simulink model "EV_longitude"  (R2024a)
settings: Solver=FixedStepAuto  StartTime=0  StopTime=inf  FixedStep=dt  RelTol=1e-3  EnableMultiTasking=on
InitFcn:
  | %open_system('EvReferenceApplication/Visualization/Performance and FE Scope');
  | dt = 0.001; %5e-5;
undefined symbols (not defined in the file): RealSimPara
libraries: autolibshared x1
settings Model: ModifiedByFormat=The MathWorks, Inc.  PauseTimes=0  Creator=The MathWorks, Inc.  LastModifiedBy=The MathWorks, Inc.
settings SolverCC: ZeroCrossAlgorithm=Adaptive  AlgebraicLoopSolver=TrustRegion  AutoInsertRateTranBlk=on  DecoupledContinuousIntegration=on  MinimalZcImpactIntegration=on
settings DataIOCC: SaveOutput=off  SignalLogging=off  DSMLogging=off  SaveTime=off
settings DebuggingCC: UnderspecifiedInitializationDetection=Classic  MergeDetectMultiDrivingBlocksExec=none  IgnoredZcDiagnostic=none  UnconnectedInputMsg=warning  UnconnectedOutputMsg=warning  UnconnectedLineMsg=warning  PregeneratedLibrarySubsystemCodeDiagnostic=none  ArithmeticOperatorsInVariantConditions=warning
settings ModelReferenceCC: UpdateModelReferenceTargets=IfOutOfDate  EnableRefExpFcnMdlSchedulingChecks=on  ModelReferenceMinAlgLoopOccurrences=on  PropagateSignalLabelsOutOfModel=off
settings SFSimCC: SimUseLocalCustomCode=off
settings RTWCC: RTWUseLocalCustomCode=off  GPUComputeCapability=3.5
settings CodeAppCC: StateflowObjectComments=on
settings GRTTargetCC: TargetLangStandard=C89/C90 (ANSI)
settings ConfigComp: CovMetricSettings=dsw  CovSaveCumulativeToWorkspaceVar=on  CovSaveSingleToWorkspaceVar=on  CovExternalEMLEnable=off

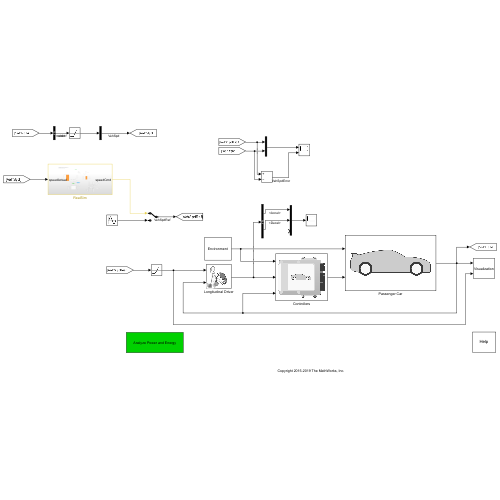
[thumbnail: Simulink's stored preview of the top-level diagram]
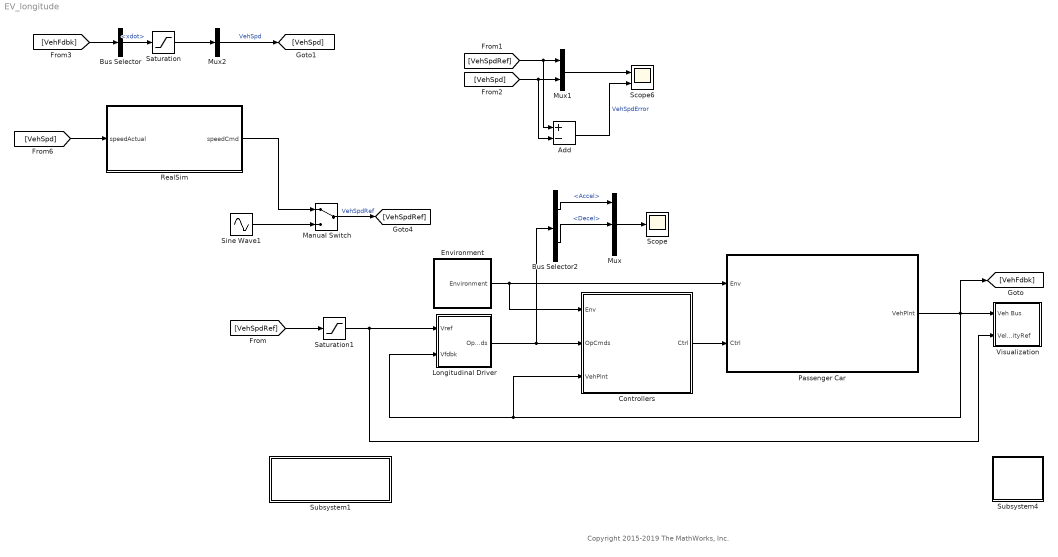
== system EV_longitude ==
  note: Copyright 2015-2019 The MathWorks, Inc.
  Add : Sum  Inputs=+-
  Bus Selector : BusSelector  OutputSignals=Veh.xdot
  Bus Selector2 : BusSelector  OutputSignals=Accel,Decel
  Controllers : Subsystem
      mask Display: image('SystemControllers.png','center')
  Environment : Subsystem
      mask Display: disp('Environment')
  Longitudinal Driver : Subsystem  Variant=on  VariantControlMode=label  VariantControl=Variant1  LabelModeActiveChoice=0  mask{tau=0.03, L=4, Kpt=10000}
      mask prompts: tau "Driver response time, tau [s]"; L "Preview distance, L [m]:"; Kpt "Effective vehicle total tractive force, Kpt [N]:"
      mask Display:
      | if strcmp('1',get_param(gcb,'ActiveVariant'))
      |     disp('Open Loop')
      | else
      |     image('LongitudinalDriver.png','center');
      | end
  Manual Switch : ManualSwitch
  Mux : Mux  Inputs=3
  Mux1 : Mux  Inputs=2
  Mux2 : Mux  Inputs=1
  Passenger Car : Subsystem
      mask Display: image('PassengerVehicle.png','center')
  RealSim : Subsystem
  Saturation : Saturate  UpperLimit=Inf  LowerLimit=0.0
  Saturation1 : Saturate  UpperLimit=Inf  LowerLimit=0.0
  Scope : Scope
  Scope6 : Scope  NumInputPorts=2
  Sine Wave1 : Sin  Bias=10  SampleTime=0
  Subsystem1 : Subsystem
      settings: OpenFcn=edit GenerateEnergyReport
      mask Display: disp('Analyze Power and Energy')
  Subsystem4 : Subsystem
      settings: OpenFcn=helpview([docroot,'/toolbox/autoblks/helptargets.map'], 'ev_refapp')
      mask Display: disp('Help')
  Visualization : Subsystem
      mask Display: disp('Visualization')
  wires:
  [VehSpdRef] -> Saturation1/1
  Environment/1(Environment) -> Controllers/1(Env), Passenger Car/1(Env)
  Controllers/1(Ctrl) -> Passenger Car/2(Ctrl)
  Mux1/1 -> Scope6/1
  Manual Switch/1 -> [VehSpdRef]  "VehSpdRef"
  [VehSpd] -> Add/2, Mux1/2
  Sine Wave1/1 -> Manual Switch/2
  RealSim/1(speedCmd) -> Manual Switch/1
  [VehSpdRef] -> Add/1, Mux1/1
  [VehSpd] -> RealSim/1(speedActual)
  Add/1 -> Scope6/2  "VehSpdError"
  Bus Selector/1 -> Saturation/1  "<xdot>"
  [VehFdbk] -> Bus Selector/1
  Passenger Car/1(VehPlnt) -> [VehFdbk], Longitudinal Driver/2("Vfdbk "), Controllers/3(VehPlnt), Visualization/1(Veh Bus)
  Bus Selector2/2 -> Mux/2  "<Decel>"
  Longitudinal Driver/1(" OpCmds") -> Bus Selector2/1, Controllers/2(OpCmds)
  Mux/1 -> Scope/1
  Bus Selector2/1 -> Mux/1  "<Accel>"
  Mux2/1 -> [VehSpd]  "VehSpd"
  Saturation/1 -> Mux2/1
  Saturation1/1 -> Visualization/2(VelocityRef), Longitudinal Driver/1("Vref ")

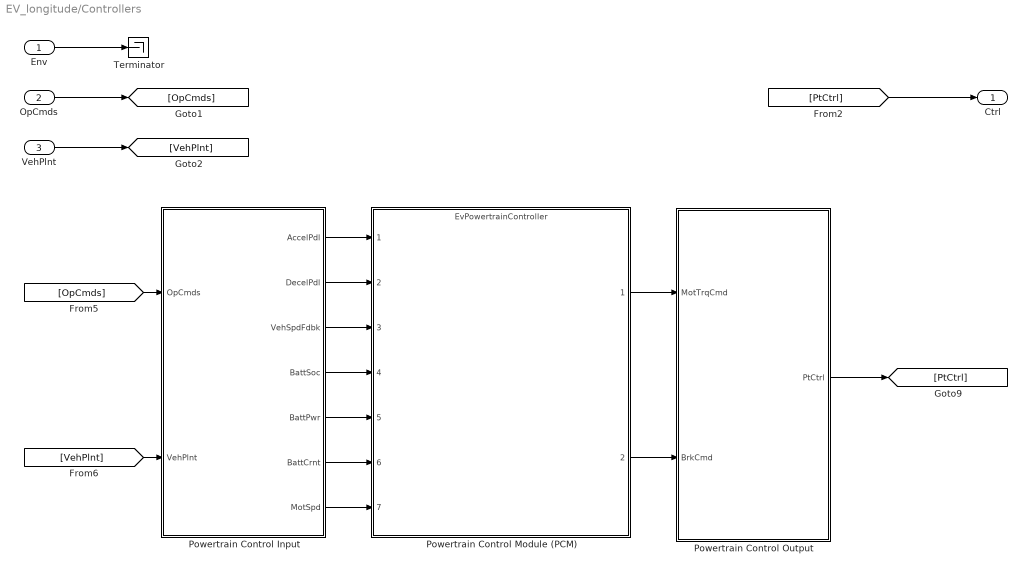
== system EV_longitude/Controllers ==
  Env : Inport
  OpCmds : Inport  Port=2
  VehPlnt : Inport  Port=3
  Powertrain Control Input : Subsystem
  Powertrain Control Module (PCM) : ModelReference  ModelNameDialog=EvPowertrainController.slx  SimulationMode=Normal  ModelReferenceVersion=1.415
  Powertrain Control Output : Subsystem
  Terminator : Terminator
  Ctrl : Outport  VectorParamsAs1DForOutWhenUnconnected=off
  wires:
  [PtCtrl] -> Ctrl/1
  Env/1 -> Terminator/1
  [OpCmds] -> Powertrain Control Input/1(OpCmds)
  Powertrain Control Output/1(PtCtrl) -> [PtCtrl]
  [VehPlnt] -> Powertrain Control Input/2(VehPlnt)
  VehPlnt/1 -> [VehPlnt]
  OpCmds/1 -> [OpCmds]
  Powertrain Control Input/4(BattSoc) -> Powertrain Control Module (PCM)/4
  Powertrain Control Input/3(VehSpdFdbk) -> Powertrain Control Module (PCM)/3
  Powertrain Control Input/2(DecelPdl) -> Powertrain Control Module (PCM)/2
  Powertrain Control Input/1(AccelPdl) -> Powertrain Control Module (PCM)/1
  Powertrain Control Input/5(BattPwr) -> Powertrain Control Module (PCM)/5
  Powertrain Control Input/6(BattCrnt) -> Powertrain Control Module (PCM)/6
  Powertrain Control Input/7(MotSpd) -> Powertrain Control Module (PCM)/7
  Powertrain Control Module (PCM)/1 -> Powertrain Control Output/1(MotTrqCmd)
  Powertrain Control Module (PCM)/2 -> Powertrain Control Output/2(BrkCmd)

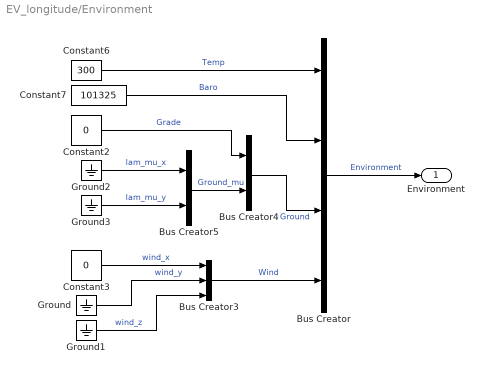
== system EV_longitude/Environment ==
  Bus Creator : BusCreator  Inputs=4
  Bus Creator3 : BusCreator  Inputs=3
  Bus Creator4 : BusCreator  Inputs=2
  Bus Creator5 : BusCreator  Inputs=2
  Constant2 : Constant  Value=0
  Constant3 : Constant  Value=0
  Constant6 : Constant  Value=300
  Constant7 : Constant  Value=101325
  Ground{,1..3} (4 alike) : Ground
  Environment : Outport  VectorParamsAs1DForOutWhenUnconnected=off
  wires:
  Ground2/1 -> Bus Creator5/1  "lam_mu_x"
  Ground3/1 -> Bus Creator5/2  "lam_mu_y"
  Bus Creator5/1 -> Bus Creator4/2  "Ground_mu"
  Bus Creator4/1 -> Bus Creator/3  "Ground"
  Bus Creator3/1 -> Bus Creator/4  "Wind"
  Constant3/1 -> Bus Creator3/1  "wind_x"
  Ground/1 -> Bus Creator3/2  "wind_y"
  Ground1/1 -> Bus Creator3/3  "wind_z"
  Constant6/1 -> Bus Creator/1  "Temp"
  Constant2/1 -> Bus Creator4/1  "Grade"
  Bus Creator/1 -> Environment/1  "Environment"
  Constant7/1 -> Bus Creator/2  "Baro"

== system EV_longitude/Longitudinal Driver ==
  note: To switch variants, right-click on this subsystem (from one level above) and chose:
      | Variant, Active choice, <your selection>
  "Vref " : Inport
  "Vfdbk " : Inport  Port=2
  Longitudinal Driver : Subsystem  VariantControl=0
      mask Display: image('LongitudinalDriver.png', 'center')
  Open Loop : Subsystem  VariantControl=1
      mask Display: disp('Open Loop')
  " OpCmds" : Outport  VectorParamsAs1DForOutWhenUnconnected=off

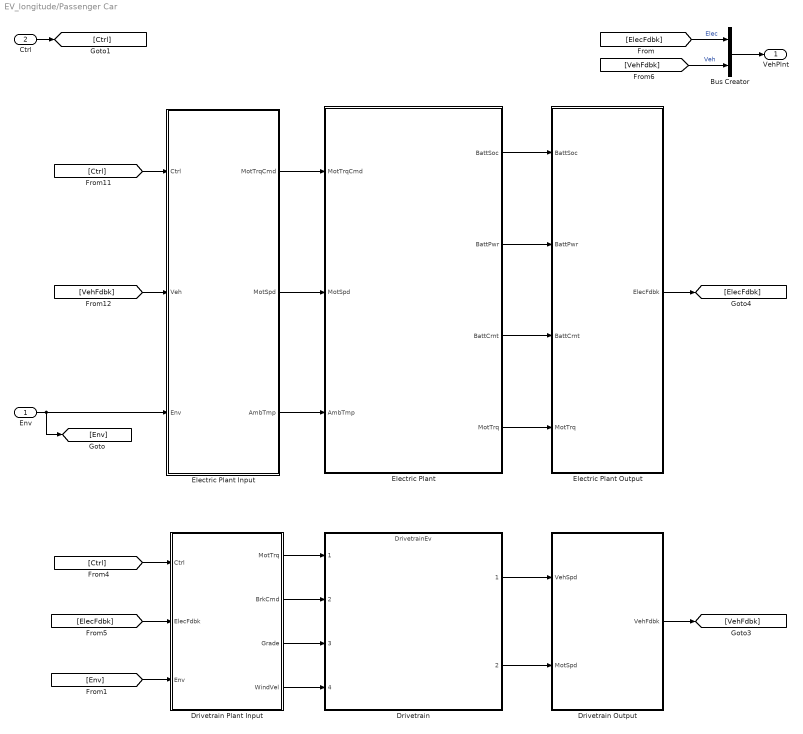
== system EV_longitude/Passenger Car ==
  Env : Inport
  Ctrl : Inport  Port=2
  Bus Creator : BusCreator  Inputs=2
  Drivetrain : ModelReference  ModelNameDialog=DrivetrainEv.slx  SimulationMode=Normal  ModelReferenceVersion=1.457
  Drivetrain Output : Subsystem
  Drivetrain Plant Input : Subsystem
  Electric Plant : Subsystem
  Electric Plant Input : Subsystem
  Electric Plant Output : Subsystem
  VehPlnt : Outport  VectorParamsAs1DForOutWhenUnconnected=off
  wires:
  Ctrl/1 -> [Ctrl]
  Env/1 -> [Env], Electric Plant Input/3(Env)
  [Ctrl] -> Drivetrain Plant Input/1(Ctrl)
  Bus Creator/1 -> VehPlnt/1
  [VehFdbk] -> Bus Creator/2  "Veh"
  Drivetrain Output/1(VehFdbk) -> [VehFdbk]
  Electric Plant Output/1(ElecFdbk) -> [ElecFdbk]
  [ElecFdbk] -> Bus Creator/1  "Elec"
  [Ctrl] -> Electric Plant Input/1(Ctrl)
  [ElecFdbk] -> Drivetrain Plant Input/2(ElecFdbk)
  [VehFdbk] -> Electric Plant Input/2(Veh)
  Drivetrain Plant Input/2(BrkCmd) -> Drivetrain/2
  Drivetrain Plant Input/1(MotTrq) -> Drivetrain/1
  Drivetrain/2 -> Drivetrain Output/2(MotSpd)
  Drivetrain/1 -> Drivetrain Output/1(VehSpd)
  Electric Plant Input/1(MotTrqCmd) -> Electric Plant/1(MotTrqCmd)
  Electric Plant Input/2(MotSpd) -> Electric Plant/2(MotSpd)
  Electric Plant/1(BattSoc) -> Electric Plant Output/1(BattSoc)
  Electric Plant/2(BattPwr) -> Electric Plant Output/2(BattPwr)
  Electric Plant/3(BattCrnt) -> Electric Plant Output/3(BattCrnt)
  Electric Plant/4(MotTrq) -> Electric Plant Output/4(MotTrq)
  Electric Plant Input/3(AmbTmp) -> Electric Plant/3(AmbTmp)
  [Env] -> Drivetrain Plant Input/3(Env)
  Drivetrain Plant Input/3(Grade) -> Drivetrain/3
  Drivetrain Plant Input/4(WindVel) -> Drivetrain/4

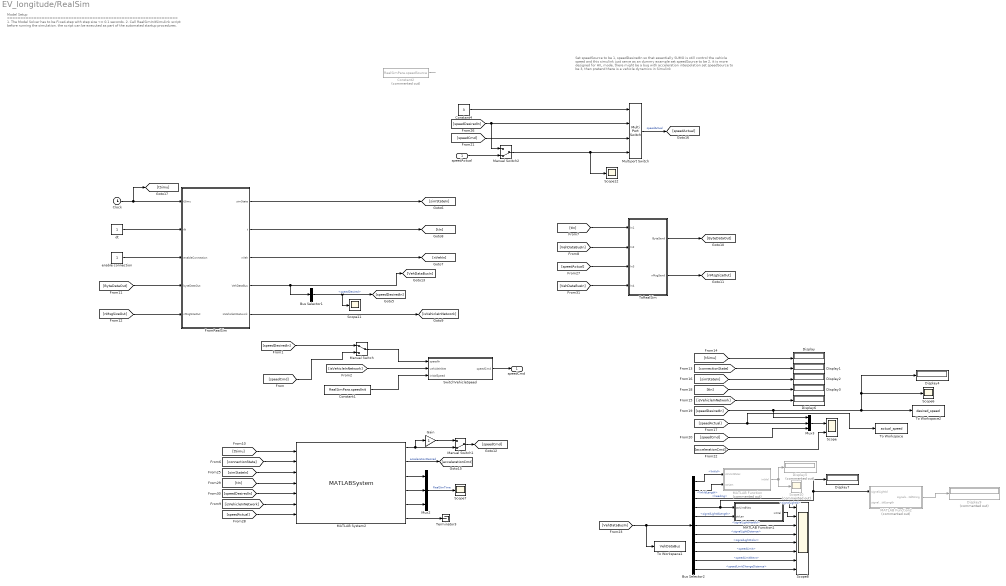
== system EV_longitude/RealSim ==
  note: Model Setup
      | ================================================================
      | 1. The Model Solver has to be Fixed-step with step size <= 0.1 seconds.
      | 2. Call RealSimInitSimulink script before running the simulation. the script can be executed as part of the automated startup procedures.
  note: Set speedSource to be 1, speedDesiredIn so that essentially SUMO is still control the vehicle speed and this simulink just serve as an dummy example
      |
      | set speedSource to be 2, it is more designed for HIL mode, there might be a bug with acceleration interpolation
      |
      | set speedSource to be 3, then pretend there is a vehicle dynamics in Simulink
  speedActual : Inport
  Bus Selector1 : BusSelector  OutputSignals=speedDesired
  Bus Selector2 : BusSelector  OutputSignals=linkId,linkIdLength,heading,signalLightId,signalLightIdLength,signalLightHeadId,signalLightDistance,signalLightColor,speedLimit,speedLimitNext,speedLimitChangeDistance
  Clock : Clock
  Constant1 : Constant  Value=RealSimPara.speedInit
  Constant2 : Constant  Commented=on  Value=RealSimPara.speedSource
  Constant4 : Constant  Value=3
  Display{,1..4,6..7} (7 alike) : Display
  Display5 : Display  Commented=on
  Display9 : Display  Commented=on
  FromRealSim : Subsystem
  Gain : Gain
  MATLAB Function : MATLAB Function  Commented=on  TreatAsAtomicUnit=on
  MATLAB Function1 : MATLAB Function  TreatAsAtomicUnit=on
  MATLAB Function2 : MATLAB Function  Commented=on  TreatAsAtomicUnit=on  SystemSampleTime=0.001
  MATLAB System2 : MATLABSystem  System=RealSimInterpSpeed  initialSpeed=RealSimPara.speedInit  speedLookAheadHorizon=RealSimPara.tLookahead  speedUpperBound=30  smoothWindow=RealSimPara.smoothWindow  SimulateUsing=Code generation
      mask Type: RealSimInterpSpeed
      mask Display:
      | disp('RealSimInterpSpeed');
      | port_label('input',1,'simulationTime');
      | port_label('input',2,'connectionState');
      | port_label('input',3,'simState');
      | port_label('input',4,'timeReceive');
      | port_label('input',5,'speedReceive');
      | port_label('input',6,'isVehicleInNetwork');
      | port_label('input',7,'speedActual');
      | port_label('output',1,'speedLookAhead');
      | port_label('output',2,'accelerationDesired');
      | port_label('output',3,'timeSimulator');
      | port_label('output',4,'timeStepSimulator');
      | port_label('output',5,'timeStepTrigger');
      | port_label('output',6,'RealSimDelay');
  Manual Switch : ManualSwitch
  Manual Switch1 : ManualSwitch  CurrentSetting=0
  Manual Switch2 : ManualSwitch  CurrentSetting=0
  Multiport Switch : MultiPortSwitch  SaturateOnIntegerOverflow=off  InputSameDT=off
  Mux2 : Mux  Inputs=3
  Mux3 : Mux  Inputs=3
  Scope : Scope  NumInputPorts=2
  Scope10 : Scope  Commented=on
  Scope{6..7,11..12} (4 alike) : Scope
  Scope8 : Scope  NumInputPorts=8
  SwitchVehicleSpeed : Subsystem
  Terminator3 : Terminator
  To Workspace : ToWorkspace  VariableName=actual_speed  SaveFormat=Timeseries  SampleTime=1
  To Workspace1 : ToWorkspace  VariableName=VehDataBus  SaveFormat=Timeseries  SampleTime=-1
  To Workspace2 : ToWorkspace  VariableName=desired_speed  SaveFormat=Timeseries  SampleTime=1
  ToRealSim : Subsystem
  dt : Constant
  enable connection : Constant
  speedCmd : Outport
  wires:
  [tSimu] -> Display/1
  Bus Selector2/5 -> MATLAB Function1/2(strLen)  "<signalLightIdLength>"
  [simStateIn] -> MATLAB System2/3
  [isVehicleInNetwork] -> Display6/1
  [ByteDataOut] -> FromRealSim/4(byteDataOut)
  MATLAB System2/5 -> Mux2/3
  [VehDataBusIn] -> To Workspace1/1, Bus Selector2/1
  MATLAB System2/1 -> Gain/1, Manual Switch1/2
  [speedCmd] -> Multiport Switch/3
  Mux2/1 -> Scope7/1  "RealSimTime"
  [tSimu] -> MATLAB System2/1
  Gain/1 -> Manual Switch1/1
  Bus Selector1/1 -> Scope11/1, [speedDesiredIn]  "<speedDesired>"
  Bus Selector2/9 -> Scope8/6  "<speedLimit>"
  [speedDesiredIn] -> Display4/1, Scope6/1, To Workspace2/1, Mux3/1
  Bus Selector2/4 -> Display7/1, MATLAB Function2/1(signalLightId), MATLAB Function1/1(strUint8Vec)  "<signalLightId>"
  MATLAB System2/3 -> Mux2/1
  dt/1 -> FromRealSim/2(dt)
  Bus Selector2/10 -> Scope8/7  "<speedLimitNext>"
  FromRealSim/4(VehDataBus) -> Bus Selector1/1, [VehDataBusIn]
  enable connection/1 -> FromRealSim/3(enableConnection)
  MATLAB Function/1(intVal) -> Scope10/1, Display5/1
  [speedDesiredIn] -> MATLAB System2/5
  [nMsgSizeOut] -> FromRealSim/5(nMsgSizeOut)
  Bus Selector2/11 -> Scope8/8  "<speedLimitChangeDistance>"
  [speedDesiredIn] -> Manual Switch2/1, Multiport Switch/2
  [speedActual] -> MATLAB System2/7
  FromRealSim/3(nVeh) -> [nVehIn]
  [speedActual] -> To Workspace/1, Mux3/2
  [connectionState] -> Display1/1
  Clock/1 -> FromRealSim/1(tSimu), [tSimu]
  [tIn] -> Display3/1
  Bus Selector2/7 -> Scope8/4  "<signalLightDistance>"
  MATLAB System2/4 -> Mux2/2
  Bus Selector2/8 -> Scope8/5  "<signalLightColor>"
  Manual Switch2/1 -> Scope12/1, Multiport Switch/4
  [connectionState] -> MATLAB System2/2
  MATLAB System2/6 -> Terminator3/1
  Bus Selector2/1 -> MATLAB Function/1(strUint8Vec)  "<linkId>"
  [tIn] -> ToRealSim/1(In1)
  MATLAB System2/2 -> [accelerationCmd]  "accelerationDesired"
  MATLAB Function2/1(signalLightIdString) -> Display9/1
  Bus Selector2/2 -> MATLAB Function/2(strLen)  "<linkIdLength>"
  [tIn] -> MATLAB System2/4
  [speedCmd] -> Mux3/3
  Constant4/1 -> Multiport Switch/1
  Manual Switch1/1 -> [speedCmd]
  ToRealSim/2(nMsgSend) -> [nMsgSizeOut]
  FromRealSim/1(simState) -> [simStateIn]
  [speedActual] -> ToRealSim/3(In3)
  FromRealSim/2(t) -> [tIn]
  FromRealSim/5(isVehicleInNetwork) -> [isVehicleInNetwork]
  [accelerationCmd] -> Scope/2
  [VehDataBusIn] -> ToRealSim/2(In2)
  Multiport Switch/1 -> [speedActual]  "speedActual"
  Bus Selector2/6 -> Scope8/3  "<signalLightHeadId>"
  [VehDataBusIn] -> ToRealSim/4(In4)
  ToRealSim/1(ByteSend) -> [ByteDataOut]
  MATLAB Function1/1(intVal) -> Scope8/2
  Bus Selector2/3 -> Scope8/1  "<heading>"
  [isVehicleInNetwork] -> MATLAB System2/6
  Mux3/1 -> Scope/1
  [simStateIn] -> Display2/1
  ? -> MATLAB Function2/2(signalLightIdLength)
  Constant2/1 -> ?
  [speedCmd] -> Manual Switch/2
  [speedDesiredIn] -> Manual Switch/1
  speedActual/1 -> Manual Switch2/2
  Constant1/1 -> SwitchVehicleSpeed/3(initialSpeed)
  [isVehicleInNetwork] -> SwitchVehicleSpeed/2(vehicleInNet)
  SwitchVehicleSpeed/1(speedCmd) -> speedCmd/1
  Manual Switch/1 -> SwitchVehicleSpeed/1(speedIn)

== system EV_longitude/Subsystem1 ==

== system EV_longitude/Subsystem4 ==

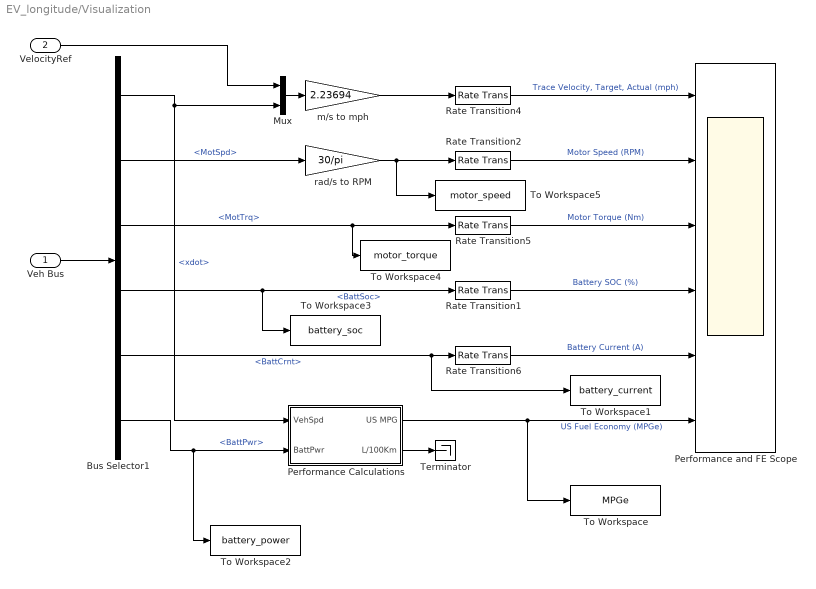
== system EV_longitude/Visualization ==
  Veh Bus : Inport
  VelocityRef : Inport  Port=2
  Bus Selector1 : BusSelector  OutputSignals=Veh.xdot,Veh.MotSpd,Elec.MotTrq,Elec.BattSoc,Elec.BattCrnt,Elec.BattPwr
  Mux : Mux  Inputs=2
  Performance Calculations : Subsystem
  Performance and FE Scope : Scope  NumInputPorts=6
  Rate Transition{1..2,4..6} (5 alike) : RateTransition  Deterministic=off
  Terminator : Terminator
  To Workspace : ToWorkspace  VariableName=MPGe  SaveFormat=Timeseries  SampleTime=1
  To Workspace1 : ToWorkspace  VariableName=battery_current  SaveFormat=Timeseries  SampleTime=1
  To Workspace2 : ToWorkspace  VariableName=battery_power  SaveFormat=Timeseries  SampleTime=1
  To Workspace3 : ToWorkspace  VariableName=battery_soc  SaveFormat=Timeseries  SampleTime=1
  To Workspace4 : ToWorkspace  VariableName=motor_torque  SaveFormat=Timeseries  SampleTime=1
  To Workspace5 : ToWorkspace  VariableName=motor_speed  SaveFormat=Timeseries  SampleTime=1
  m/s to mph : Gain  Gain=2.23694
  rad/s to RPM : Gain  Gain=30/pi
  wires:
  Veh Bus/1 -> Bus Selector1/1
  Bus Selector1/1 -> Performance Calculations/1(VehSpd), Mux/2  "<xdot>"
  Mux/1 -> m/s to mph/1
  Performance Calculations/1(US MPG) -> To Workspace/1, Performance and FE Scope/6  "US Fuel Economy (MPGe)"
  Performance Calculations/2(L/100Km) -> Terminator/1
  m/s to mph/1 -> Rate Transition4/1
  Bus Selector1/4 -> To Workspace3/1, Rate Transition1/1  "<BattSoc>"
  VelocityRef/1 -> Mux/1
  Rate Transition1/1 -> Performance and FE Scope/4  "Battery SOC (%)"
  Rate Transition2/1 -> Performance and FE Scope/2  "Motor Speed (RPM)"
  Rate Transition4/1 -> Performance and FE Scope/1  "Trace Velocity, Target, Actual (mph)"
  Bus Selector1/2 -> rad/s to RPM/1  "<MotSpd>"
  Bus Selector1/6 -> To Workspace2/1, Performance Calculations/2(BattPwr)  "<BattPwr>"
  rad/s to RPM/1 -> To Workspace5/1, Rate Transition2/1
  Bus Selector1/3 -> To Workspace4/1, Rate Transition5/1  "<MotTrq>"
  Rate Transition5/1 -> Performance and FE Scope/3  "Motor Torque (Nm)"
  Rate Transition6/1 -> Performance and FE Scope/5  "Battery Current (A)"
  Bus Selector1/5 -> To Workspace1/1, Rate Transition6/1  "<BattCrnt>"

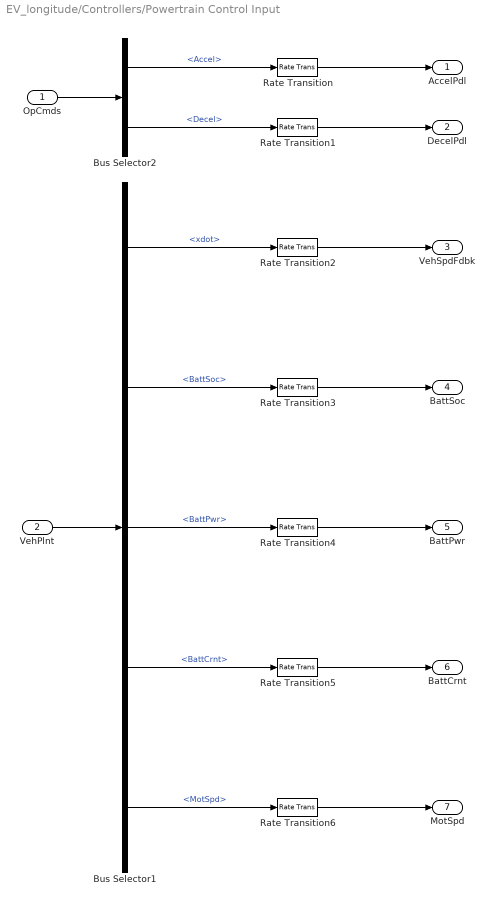
== system EV_longitude/Controllers/Powertrain Control Input ==
  OpCmds : Inport
  VehPlnt : Inport  Port=2
  Bus Selector1 : BusSelector  OutputSignals=Veh.xdot,Elec.BattSoc,Elec.BattPwr,Elec.BattCrnt,Veh.MotSpd
  Bus Selector2 : BusSelector  OutputSignals=Accel,Decel
  Rate Transition{,1..6} (7 alike) : RateTransition  Deterministic=off
  AccelPdl : Outport  VectorParamsAs1DForOutWhenUnconnected=off
  DecelPdl : Outport  Port=2  VectorParamsAs1DForOutWhenUnconnected=off
  VehSpdFdbk : Outport  Port=3  VectorParamsAs1DForOutWhenUnconnected=off
  BattSoc : Outport  Port=4  VectorParamsAs1DForOutWhenUnconnected=off
  BattPwr : Outport  Port=5  VectorParamsAs1DForOutWhenUnconnected=off
  BattCrnt : Outport  Port=6  VectorParamsAs1DForOutWhenUnconnected=off
  MotSpd : Outport  Port=7  VectorParamsAs1DForOutWhenUnconnected=off
  wires:
  OpCmds/1 -> Bus Selector2/1
  VehPlnt/1 -> Bus Selector1/1
  Bus Selector2/1 -> Rate Transition/1  "<Accel>"
  Bus Selector2/2 -> Rate Transition1/1  "<Decel>"
  Bus Selector1/1 -> Rate Transition2/1  "<xdot>"
  Bus Selector1/2 -> Rate Transition3/1  "<BattSoc>"
  Bus Selector1/3 -> Rate Transition4/1  "<BattPwr>"
  Bus Selector1/4 -> Rate Transition5/1  "<BattCrnt>"
  Bus Selector1/5 -> Rate Transition6/1  "<MotSpd>"
  Rate Transition/1 -> AccelPdl/1
  Rate Transition1/1 -> DecelPdl/1
  Rate Transition2/1 -> VehSpdFdbk/1
  Rate Transition3/1 -> BattSoc/1
  Rate Transition4/1 -> BattPwr/1
  Rate Transition5/1 -> BattCrnt/1
  Rate Transition6/1 -> MotSpd/1

== system EV_longitude/Controllers/Powertrain Control Output ==
  MotTrqCmd : Inport
  BrkCmd : Inport  Port=2
  Bus Creator : BusCreator  Inputs=2
  PtCtrl : Outport  VectorParamsAs1DForOutWhenUnconnected=off
  wires:
  BrkCmd/1 -> Bus Creator/2  "BrkCmd"
  Bus Creator/1 -> PtCtrl/1  "PtCtrl"
  MotTrqCmd/1 -> Bus Creator/1  "MotTrqCmd"

== system EV_longitude/Longitudinal Driver/Longitudinal Driver ==
  Vref : Inport
  Vfdbk : Inport  Port=2
  Bus Selector : BusSelector  OutputSignals=Veh.xdot
  Ground : Ground
  Longitudinal Driver Model : autolibshared/Longitudinal Driver  extAccelOvr=off  extDecelOvr=off  extAccelHld=off  extDecelHld=off  extAccelZero=off  extDecelZero=off  cntrlType=Predictive  shftType=Reverse, Neutral, Drive  velUnits=m/s  gearOut=off  Kp=1  Ki=1  Kff=0  Kg=0  VehVelVec=[0 100]  KffVec=[.1 .1]  KpVec=[10 10]  KiVec=[5 5]  KgVec=[0 0]  m=1500  Kpt=Kpt  tau=tau  L=L  aR=160  bR=1  cR=0.36  g=9.81  vnom=1  Kaw=0  tauerr=0  tauPt=2  GearInit=0  tShift=.1  pdlVec=[0.1 0.4 0.5 0.9]  upShftTbl=[-1 12.9375 26.4375 39.9375 51.18749999999999 62.4375 72.84375 83.25;-1 16.3125 29.8125 43.3125 54.5624 65.8125 76.78125 87.75;-1 19.6875 33.1875 46.68749999999999 57.9375 69.1875 80.71875 92.25;-1 33 52.5 77.25 100.5 138.75 161.875 185]  dwnShftTbl=[1 9.5625 23.0625 36.5625 47.8125 59.0625 68.90625 78.75;1 12.9375 26.4375 39.9375 51.18749999999999 62.4375 72.84375 83.25;1 16.3125 29.8125 43.3125 54.562499 65.8125 76.78125 87.75;1 19.6875 33.1875 46.68749999999999 57.9375 69.1875 80.71875 92.25]  tClutch=.5  tRev=.5  tPark=120  aMode=1  UpGearVec="[0  1  2  3  4  5  6  7]"  DownGearVec="[1  2  3  4  5  6  7  8]"
  Terminator : Terminator
  Terminator1 : Terminator
  OpCmds : Outport  VectorParamsAs1DForOutWhenUnconnected=off
  wires:
  Bus Selector/1 -> Longitudinal Driver Model/2  "<xdot>"
  Vref/1 -> Longitudinal Driver Model/1  "xdotref"
  Vfdbk/1 -> Bus Selector/1
  Longitudinal Driver Model/2 -> Terminator/1  "Acc"
  Longitudinal Driver Model/3 -> Terminator1/1  "Dec"
  Ground/1 -> Longitudinal Driver Model/3
  Longitudinal Driver Model/1 -> OpCmds/1  "Info"

== system EV_longitude/Longitudinal Driver/Open Loop ==
  note: This subsystem is provided to disable the driver subsystem and expose the driver interface.
      |
      | The interface can:
      | - be connected with dashboard UI blocks or 3rd party hardware
      | - provide application specific pre-programmed event or time based signals
      | - be driven by recorded operator signals for tuning, troubleshooting and model validation
  Bus Creator2 : BusCreator  Inputs=8
  Constant{1..4} (4 alike) : Constant  Value=0
  Ground{,1..3} (4 alike) : Ground
  OpCmds : Outport  VectorParamsAs1DForOutWhenUnconnected=off
  wires:
  Ground3/1 -> Bus Creator2/8  "ErrMin"
  Ground1/1 -> Bus Creator2/6  "ErrSqrSum"
  Bus Creator2/1 -> OpCmds/1  "Info"
  Ground2/1 -> Bus Creator2/7  "ErrMax"
  Constant1/1 -> Bus Creator2/1  "Accel"
  Constant3/1 -> Bus Creator2/3  "Gear"
  Constant2/1 -> Bus Creator2/2  "Decel"
  Ground/1 -> Bus Creator2/5  "Err"
  Constant4/1 -> Bus Creator2/4  "Clutch"

== system EV_longitude/Passenger Car/Drivetrain Output ==
  VehSpd : Inport
  MotSpd : Inport  Port=2
  Bus Creator1 : BusCreator  Inputs=2
  VehFdbk : Outport  VectorParamsAs1DForOutWhenUnconnected=off
  wires:
  Bus Creator1/1 -> VehFdbk/1  "VehFdbk"
  VehSpd/1 -> Bus Creator1/1
  MotSpd/1 -> Bus Creator1/2  "MotSpd"

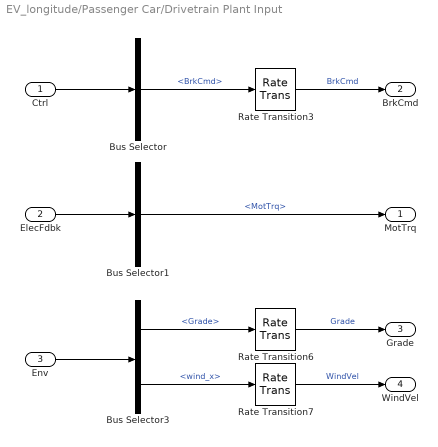
== system EV_longitude/Passenger Car/Drivetrain Plant Input ==
  Ctrl : Inport
  ElecFdbk : Inport  Port=2
  Env : Inport  Port=3
  Bus Selector : BusSelector  OutputSignals=BrkCmd
  Bus Selector1 : BusSelector  OutputSignals=MotTrq
  Bus Selector3 : BusSelector  OutputSignals=Ground.Grade,Wind.wind_x
  Rate Transition3 : RateTransition  Deterministic=off
  Rate Transition6 : RateTransition  Deterministic=off
  Rate Transition7 : RateTransition  Deterministic=off
  MotTrq : Outport  VectorParamsAs1DForOutWhenUnconnected=off
  BrkCmd : Outport  Port=2  VectorParamsAs1DForOutWhenUnconnected=off
  Grade : Outport  Port=3  VectorParamsAs1DForOutWhenUnconnected=off
  WindVel : Outport  Port=4  VectorParamsAs1DForOutWhenUnconnected=off
  wires:
  Ctrl/1 -> Bus Selector/1
  Bus Selector/1 -> Rate Transition3/1  "<BrkCmd>"
  Rate Transition3/1 -> BrkCmd/1  "BrkCmd"
  ElecFdbk/1 -> Bus Selector1/1
  Bus Selector1/1 -> MotTrq/1  "<MotTrq>"
  Env/1 -> Bus Selector3/1
  Rate Transition6/1 -> Grade/1  "Grade"
  Rate Transition7/1 -> WindVel/1  "WindVel"
  Bus Selector3/1 -> Rate Transition6/1  "<Grade>"
  Bus Selector3/2 -> Rate Transition7/1  "<wind_x>"

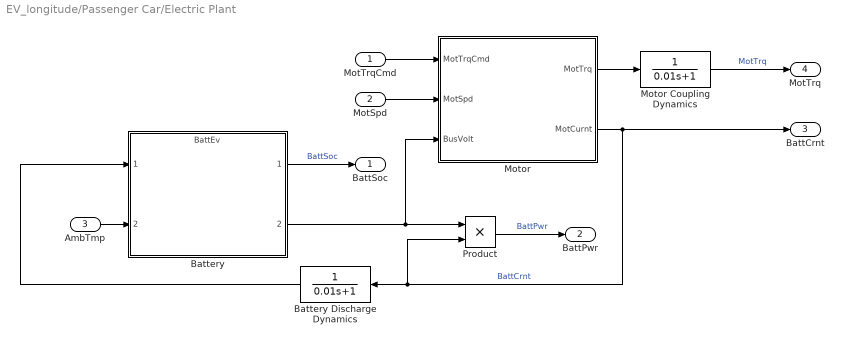
== system EV_longitude/Passenger Car/Electric Plant ==
  MotTrqCmd : Inport
  MotSpd : Inport  Port=2
  AmbTmp : Inport  Port=3
  Battery : ModelReference  ModelNameDialog=BattEv.slx  SimulationMode=Normal  ModelReferenceVersion=1.706
  Battery Discharge Dynamics : TransferFcn  Denominator=[0.01 1]
  Motor : Subsystem  Variant=on  VariantControlMode=label  LabelModeActiveChoice=MotGenEvMapped
  Motor Coupling Dynamics : TransferFcn  Denominator=[0.01 1]
  Product : Product
  BattSoc : Outport  VectorParamsAs1DForOutWhenUnconnected=off
  BattPwr : Outport  Port=2  VectorParamsAs1DForOutWhenUnconnected=off
  BattCrnt : Outport  Port=3  VectorParamsAs1DForOutWhenUnconnected=off
  MotTrq : Outport  Port=4  VectorParamsAs1DForOutWhenUnconnected=off
  wires:
  MotTrqCmd/1 -> Motor/1(MotTrqCmd)
  MotSpd/1 -> Motor/2(MotSpd)
  AmbTmp/1 -> Battery/2
  Battery/1 -> BattSoc/1  "BattSoc"
  Battery/2 -> Motor/3(BusVolt), Product/1
  Product/1 -> BattPwr/1  "BattPwr"
  Motor/2(MotCurnt) -> Battery Discharge Dynamics/1, Product/2, BattCrnt/1  "BattCrnt"
  Battery Discharge Dynamics/1 -> Battery/1
  Motor/1(MotTrq) -> Motor Coupling Dynamics/1
  Motor Coupling Dynamics/1 -> MotTrq/1  "MotTrq"

== system EV_longitude/Passenger Car/Electric Plant Input ==
  Ctrl : Inport
  Veh : Inport  Port=2
  Env : Inport  Port=3
  Bus Selector : BusSelector  OutputSignals=MotTrqCmd
  Bus Selector1 : BusSelector  OutputSignals=MotSpd
  Bus Selector2 : BusSelector  OutputSignals=Temp
  Rate Transition1 : RateTransition  Deterministic=off
  Rate Transition5 : RateTransition  Deterministic=off
  MotTrqCmd : Outport  VectorParamsAs1DForOutWhenUnconnected=off
  MotSpd : Outport  Port=2  VectorParamsAs1DForOutWhenUnconnected=off
  AmbTmp : Outport  Port=3  VectorParamsAs1DForOutWhenUnconnected=off
  wires:
  Rate Transition5/1 -> MotTrqCmd/1  "MotTrqCmd"
  Ctrl/1 -> Bus Selector/1
  Bus Selector/1 -> Rate Transition5/1  "<MotTrqCmd>"
  Veh/1 -> Bus Selector1/1
  Bus Selector1/1 -> MotSpd/1  "<MotSpd>"
  Env/1 -> Bus Selector2/1
  Rate Transition1/1 -> AmbTmp/1  "AmbTmp"
  Bus Selector2/1 -> Rate Transition1/1  "<Temp>"

== system EV_longitude/Passenger Car/Electric Plant Output ==
  BattSoc : Inport
  BattPwr : Inport  Port=2
  BattCrnt : Inport  Port=3
  MotTrq : Inport  Port=4
  Bus Creator1 : BusCreator  Inputs=4
  ElecFdbk : Outport  VectorParamsAs1DForOutWhenUnconnected=off
  wires:
  Bus Creator1/1 -> ElecFdbk/1  "ElecFdbk"
  BattPwr/1 -> Bus Creator1/2
  BattSoc/1 -> Bus Creator1/1
  BattCrnt/1 -> Bus Creator1/3
  MotTrq/1 -> Bus Creator1/4

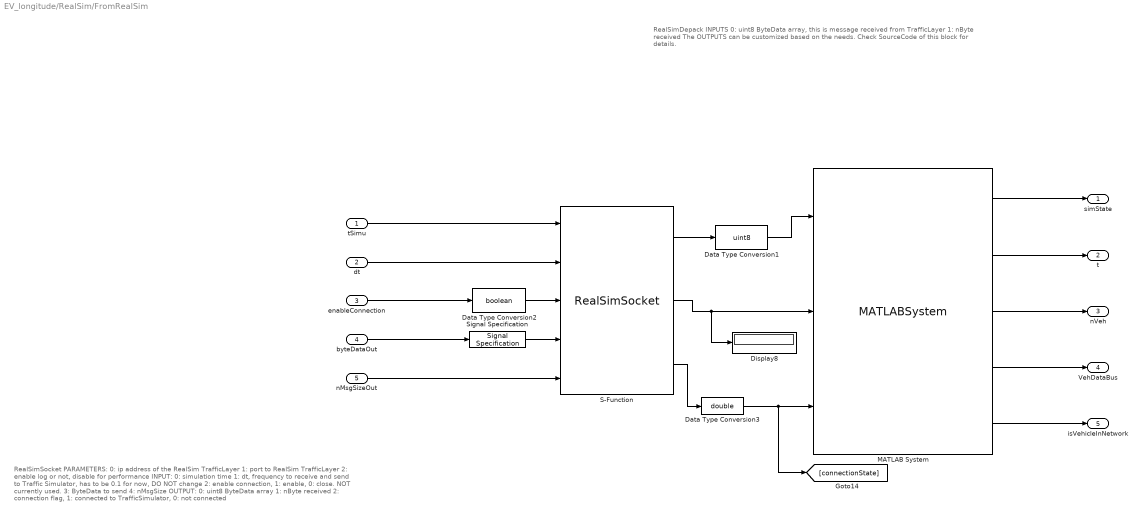
== system EV_longitude/RealSim/FromRealSim ==
  note: RealSimSocket
      | PARAMETERS:
      | 0: ip address of the RealSim TrafficLayer
      | 1: port to RealSim TrafficLayer
      | 2: enable log or not, disable for performance
      | INPUT:
      | 0: simulation time
      | 1: dt, frequency to receive and send to Traffic Simulator, has to be 0.1 for now, DO NOT change
      | 2: enable connection, 1: enable, 0: close. NOT currently used.
      | 3: ByteData to send
      | 4: nMsgSize
      |
      | OUTPUT:
      | 0: uint8 ByteData array
      | 1: nByte received
      | 2: connection flag, 1: connected to TrafficSimulator, 0: not connected
  note: RealSimDepack
      | INPUTS
      | 0: uint8 ByteData array, this is message received from TrafficLayer
      | 1: nByte received
      |
      | The OUTPUTS can be customized based on the needs. Check SourceCode of this block for details.
  tSimu : Inport
  dt : Inport  Port=2
  enableConnection : Inport  Port=3
  byteDataOut : Inport  Port=4
  nMsgSizeOut : Inport  Port=5
  Data Type Conversion1 : DataTypeConversion  OutDataTypeStr=uint8  SaturateOnIntegerOverflow=off  RndMeth=Floor
  Data Type Conversion2 : DataTypeConversion  OutDataTypeStr=boolean  SaturateOnIntegerOverflow=off  RndMeth=Floor
  Data Type Conversion3 : DataTypeConversion  OutDataTypeStr=double  SaturateOnIntegerOverflow=off  RndMeth=Floor
  Display8 : Display
  MATLAB System : MATLABSystem  System=RealSimDepack  OutputBusName=VehDataBus  VehicleMessageFieldDefInputVec=VehicleMessageFieldDefInputVec  SimulateUsing=Code generation
      mask Type: RealSimDepack
      mask Display:
      | disp('RealSimDepack');
      | port_label('input',1,'ByteData');
      | port_label('input',2,'nByte');
      | port_label('input',3,'connectionState');
      | port_label('output',1,'simState');
      | port_label('output',2,'t');
      | port_label('output',3,'nVeh');
      | port_label('output',4,'VehDataBus');
      | port_label('output',5,'isVehicleInNetwork');
  S-Function : S-Function  FunctionName=RealSimSocket  Parameters=TrafficLayerIP, TrafficLayerPort, 0  SFunctionDeploymentMode=off  EnableBusSupport=off
  Signal Specification : SignalSpecification  Dimensions=[200 1]
  simState : Outport
  t : Outport  Port=2
  nVeh : Outport  Port=3
  VehDataBus : Outport  Port=4
  isVehicleInNetwork : Outport  Port=5
  wires:
  nMsgSizeOut/1 -> S-Function/5
  Data Type Conversion3/1 -> [connectionState], MATLAB System/3
  S-Function/3 -> Data Type Conversion3/1
  MATLAB System/2 -> t/1
  byteDataOut/1 -> Signal Specification/1
  Data Type Conversion1/1 -> MATLAB System/1
  S-Function/2 -> Display8/1, MATLAB System/2
  Signal Specification/1 -> S-Function/4
  Data Type Conversion2/1 -> S-Function/3
  S-Function/1 -> Data Type Conversion1/1
  MATLAB System/4 -> VehDataBus/1
  MATLAB System/1 -> simState/1
  MATLAB System/3 -> nVeh/1
  MATLAB System/5 -> isVehicleInNetwork/1
  tSimu/1 -> S-Function/1
  dt/1 -> S-Function/2
  enableConnection/1 -> Data Type Conversion2/1

== system EV_longitude/RealSim/SwitchVehicleSpeed ==
  speedIn : Inport
  vehicleInNet : Inport  Port=2
  initialSpeed : Inport  Port=3
  Switch : Switch  Criteria=u2 > Threshold  SaturateOnIntegerOverflow=off  InputSameDT=off
  speedCmd : Outport
  wires:
  Switch/1 -> speedCmd/1
  speedIn/1 -> Switch/1
  vehicleInNet/1 -> Switch/2
  initialSpeed/1 -> Switch/3

== system EV_longitude/RealSim/ToRealSim ==
  note: RealSimPack
      | INPUTS
      | 1. simState: always set to 1. NOT actively used.
      | 2. t: simulation time
      | 3. speedDesired: desired speed in m/s, For Toyota, leave as 0.
      | 4. accelerationDesired: desired acceleration in m/s^2
      | 5. id: string of the vehicle id, will be received from RealSimDepack and as one of its output.
      | 6. idLength: length of the vehicle id string, will be received from RealSimDepack and as one of its outputs
      | 7: activeLaneChange: activeLaneChange command, 0: no lane change, +1: change to left lane, -1: change to right lane. NOTE: need to reset activeLaneChange to 0 after lane change finishes, otherwise vehicle will keep making lane change. Will receive 0 activeLaneChangeFdbk from RealSimDepack when lane change finishes.
      |
      | NOTE 1: Currently, only speedDesired and/or accelerationDesired can be sent to VISSIM/SUMO. The data format receive and send are the same so other mesage fields of the send data are irrelevant and can be set to empty or zero.
      |
      | NOTE 2: if select both speedDesired and accelerationDesired
      | in config.yaml, then only accelerationDesired will be used
      | to control vehicles in TrafficSimulator. if only one of
      | speedDesired and accelerationDesired selected in
      | config.yaml, then the one selected will be used for
      | control, the other input can be leave as 0.
      |
      | NOTE 3: for VISSIM, speedDesired or accelerationDesired will be the control command 0.2 seconds in the future.
      |
      | OUTPUTS
      | 1.ByteData: bytes vector that will be sent to TrafficSimualtor
      | 2.nMsgSize: size of bytes to be sent
  In1 : Inport
  In2 : Inport  Port=2
  In3 : Inport  Port=3
  In4 : Inport  Port=4
  Bus Selector3 : BusSelector  OutputSignals=accelerationDesired
  MATLAB System1 : MATLABSystem  System=RealSimPack  VehicleMessageFieldDefInputVec=VehicleMessageFieldDefInputVec  SimulateUsing=Code generation
      mask Type: RealSimPack
      mask Display:
      | disp('RealSimPack');
      | port_label('input',1,'simState');
      | port_label('input',2,'t');
      | port_label('input',3,'VehDataBus');
      | port_label('output',1,'ByteData');
      | port_label('output',2,'nMsgSize');
  RealSim CreatBus : Subsystem
  activeLaneChange : Constant  Value=0
  rgba : Constant  Value=[255,0,0,255]
  simState : Constant
  ByteSend : Outport
  nMsgSend : Outport  Port=2
  wires:
  rgba/1 -> RealSim CreatBus/3(color)
  MATLAB System1/2 -> nMsgSend/1  "nMsgSend"
  In3/1 -> RealSim CreatBus/2(speedDesired)
  In1/1 -> MATLAB System1/2
  simState/1 -> MATLAB System1/1
  Bus Selector3/1 -> RealSim CreatBus/4(accelerationDesired)  "<accelerationDesired>"
  RealSim CreatBus/1(Out) -> MATLAB System1/3
  activeLaneChange/1 -> RealSim CreatBus/5(activeLaneChange)
  MATLAB System1/1 -> ByteSend/1  "ByteSend"
  In4/1 -> Bus Selector3/1
  In2/1 -> RealSim CreatBus/1(In)

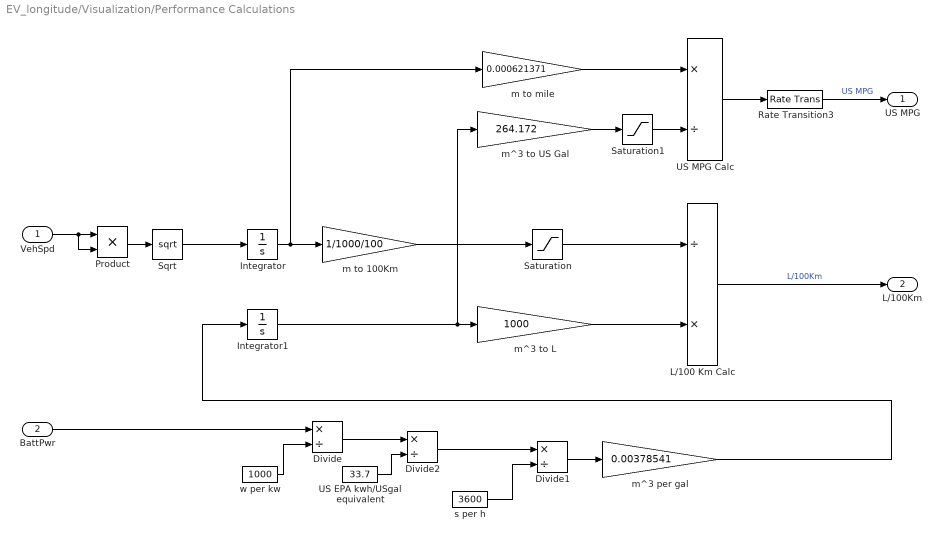
== system EV_longitude/Visualization/Performance Calculations ==
  VehSpd : Inport
  BattPwr : Inport  Port=2
  Divide : Product  Inputs=*/
  Divide1 : Product  Inputs=*/
  Divide2 : Product  Inputs=*/
  Integrator : Integrator
  Integrator1 : Integrator
  L/100 Km Calc : Product  Inputs=/*
  Product : Product
  Rate Transition3 : RateTransition  Deterministic=off
  Saturation : Saturate  UpperLimit=Inf  LowerLimit=0.001
  Saturation1 : Saturate  UpperLimit=Inf  LowerLimit=1e-3
  Sqrt : Sqrt
  US EPA kwh/USgal equivalent : Constant  Value=33.7
  US MPG Calc : Product  Inputs=*/
  m to 100Km : Gain  Gain=1/1000/100
  m to mile : Gain  Gain=0.000621371
  m^3 per gal : Gain  Gain=0.00378541
  m^3 to L : Gain  Gain=1000
  m^3 to US Gal : Gain  Gain=264.172
  s per h : Constant  Value=3600
  w per kw : Constant  Value=1000
  US MPG : Outport  VectorParamsAs1DForOutWhenUnconnected=off
  L/100Km : Outport  Port=2  VectorParamsAs1DForOutWhenUnconnected=off
  wires:
  m^3 to US Gal/1 -> Saturation1/1
  m^3 to L/1 -> L/100 Km Calc/2
  Integrator/1 -> m to mile/1, m to 100Km/1
  m to mile/1 -> US MPG Calc/1
  Integrator1/1 -> m^3 to US Gal/1, m^3 to L/1
  Saturation/1 -> L/100 Km Calc/1
  m to 100Km/1 -> Saturation/1
  L/100 Km Calc/1 -> L/100Km/1  "L/100Km"
  US MPG Calc/1 -> Rate Transition3/1
  Saturation1/1 -> US MPG Calc/2
  Rate Transition3/1 -> US MPG/1  "US MPG"
  w per kw/1 -> Divide/2
  Divide/1 -> Divide2/1
  Divide2/1 -> Divide1/1
  s per h/1 -> Divide1/2
  Divide1/1 -> m^3 per gal/1
  m^3 per gal/1 -> Integrator1/1
  US EPA kwh/USgal equivalent/1 -> Divide2/2
  BattPwr/1 -> Divide/1
  Sqrt/1 -> Integrator/1
  Product/1 -> Sqrt/1
  VehSpd/1 -> Product/2, Product/1

== system EV_longitude/Passenger Car/Electric Plant/Motor ==
  MotTrqCmd : Inport
  MotSpd : Inport  Port=2
  BusVolt : Inport  Port=3
  MotGenEvDynamic : ModelReference  ModelNameDialog=MotGenEvDynamic.slx  SimulationMode=Normal  VariantControl=MotGenEvDynamic  ModelReferenceVersion=1.356
  MotGenEvMapped : ModelReference  ModelNameDialog=MotGenEvMapped.slx  SimulationMode=Normal  VariantControl=MotGenEvMapped  ModelReferenceVersion=1.354
  MotTrq : Outport  VectorParamsAs1DForOutWhenUnconnected=off
  MotCurnt : Outport  Port=2  VectorParamsAs1DForOutWhenUnconnected=off

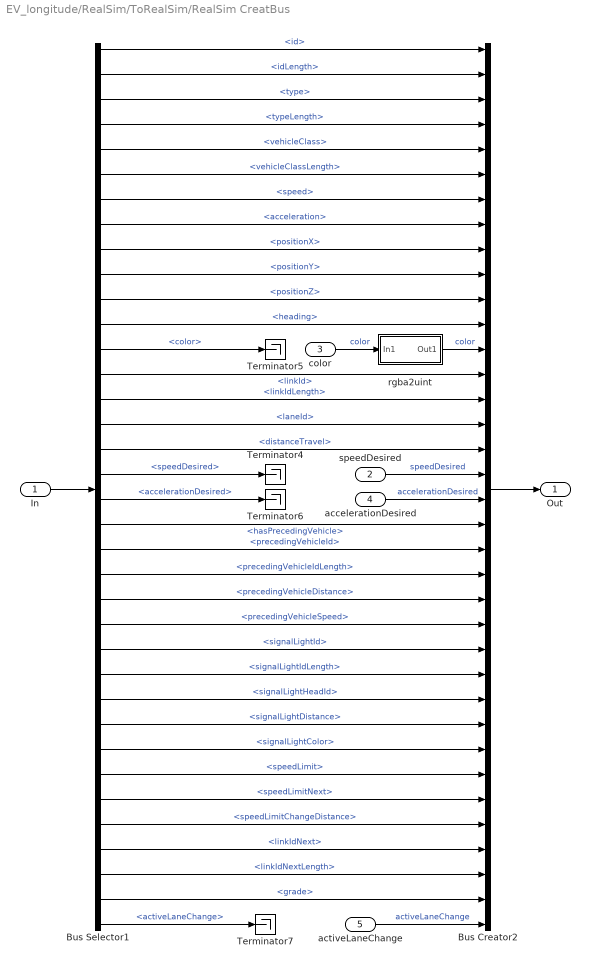
== system EV_longitude/RealSim/ToRealSim/RealSim CreatBus ==
  In : Inport
  speedDesired : Inport  Port=2
  color : Inport  Port=3
  accelerationDesired : Inport  Port=4
  activeLaneChange : Inport  Port=5
  Bus Creator2 : BusCreator  Inputs=36  OutDataTypeStr=Bus: VehDataBus
  Bus Selector1 : BusSelector  OutputSignals=id,idLength,type,typeLength,vehicleClass,vehicleClassLength,speed,acceleration,positionX,positionY,positionZ,heading,color,linkId,linkIdLength,laneId,distanceTravel,speedDesired,accelerationDesired,hasPrecedingVehicle,precedingVehicleId,precedingVehicleIdLength,precedingVehicleDistance,precedingVehicleSpeed,signalLightId,signalLightIdLength,signalLightHeadId,signalLightDistance,signalLightColor,speedLimit,speedLimitNext,speedLimitChangeDistance,linkIdNext,linkIdNextLength,grade,activeLaneChange
  Terminator{4..7} (4 alike) : Terminator
  rgba2uint : Subsystem
  Out : Outport
  wires:
  In/1 -> Bus Selector1/1
  Bus Selector1/1 -> Bus Creator2/1  "<id>"
  Bus Selector1/2 -> Bus Creator2/2  "<idLength>"
  Bus Selector1/3 -> Bus Creator2/3  "<type>"
  Bus Selector1/4 -> Bus Creator2/4  "<typeLength>"
  Bus Selector1/5 -> Bus Creator2/5  "<vehicleClass>"
  Bus Selector1/6 -> Bus Creator2/6  "<vehicleClassLength>"
  Bus Selector1/7 -> Bus Creator2/7  "<speed>"
  Bus Selector1/8 -> Bus Creator2/8  "<acceleration>"
  Bus Selector1/9 -> Bus Creator2/9  "<positionX>"
  Bus Selector1/10 -> Bus Creator2/10  "<positionY>"
  Bus Selector1/11 -> Bus Creator2/11  "<positionZ>"
  Bus Selector1/12 -> Bus Creator2/12  "<heading>"
  Bus Selector1/13 -> Terminator5/1  "<color>"
  Bus Selector1/14 -> Bus Creator2/14  "<linkId>"
  Bus Selector1/15 -> Bus Creator2/15  "<linkIdLength>"
  Bus Selector1/16 -> Bus Creator2/16  "<laneId>"
  Bus Selector1/17 -> Bus Creator2/17  "<distanceTravel>"
  Bus Selector1/18 -> Terminator4/1  "<speedDesired>"
  Bus Selector1/19 -> Terminator6/1  "<accelerationDesired>"
  Bus Selector1/20 -> Bus Creator2/20  "<hasPrecedingVehicle>"
  Bus Selector1/21 -> Bus Creator2/21  "<precedingVehicleId>"
  Bus Selector1/22 -> Bus Creator2/22  "<precedingVehicleIdLength>"
  Bus Selector1/23 -> Bus Creator2/23  "<precedingVehicleDistance>"
  Bus Selector1/24 -> Bus Creator2/24  "<precedingVehicleSpeed>"
  Bus Selector1/25 -> Bus Creator2/25  "<signalLightId>"
  Bus Selector1/26 -> Bus Creator2/26  "<signalLightIdLength>"
  Bus Selector1/27 -> Bus Creator2/27  "<signalLightHeadId>"
  Bus Selector1/28 -> Bus Creator2/28  "<signalLightDistance>"
  Bus Selector1/29 -> Bus Creator2/29  "<signalLightColor>"
  Bus Selector1/30 -> Bus Creator2/30  "<speedLimit>"
  Bus Selector1/31 -> Bus Creator2/31  "<speedLimitNext>"
  Bus Selector1/32 -> Bus Creator2/32  "<speedLimitChangeDistance>"
  Bus Selector1/33 -> Bus Creator2/33  "<linkIdNext>"
  Bus Selector1/34 -> Bus Creator2/34  "<linkIdNextLength>"
  Bus Selector1/35 -> Bus Creator2/35  "<grade>"
  Bus Selector1/36 -> Terminator7/1  "<activeLaneChange>"
  activeLaneChange/1 -> Bus Creator2/36  "activeLaneChange"
  speedDesired/1 -> Bus Creator2/18  "speedDesired"
  accelerationDesired/1 -> Bus Creator2/19  "accelerationDesired"
  color/1 -> rgba2uint/1(In1)  "color"
  rgba2uint/1(Out1) -> Bus Creator2/13  "color"
  Bus Creator2/1 -> Out/1

== system EV_longitude/RealSim/ToRealSim/RealSim CreatBus/rgba2uint ==
  In1 : Inport
  Divide : Product  Inputs=**
  Sum of Elements : Sum  Inputs=+
  rgba bit operation : Constant  Value=[2^24,2^16,2^8,2^0]
  Out1 : Outport
  wires:
  Divide/1 -> Sum of Elements/1
  In1/1 -> Divide/1
  rgba bit operation/1 -> Divide/2
  Sum of Elements/1 -> Out1/1

== matlab function EV_longitude/RealSim/MATLAB Function1 ==
  data: strUint8Vec input; intVal output double; strLen input
function intVal = strVec2Int(strUint8Vec, strLen)

    strVec = blanks(50);
    for i = 1:strLen
       strVec(i) = strUint8Vec(i); 
    end
    if strLen > 0
        intVal = real(str2double(strVec(1:strLen)));
    else
        intVal = -1;
    end

== matlab function EV_longitude/RealSim/MATLAB Function2 ==
  data: signalLightId input uint8 size=[1 50]; signalLightIdString output string; signalLightIdLength input
function signalLightIdString = fcn(signalLightId, signalLightIdLength)

signalLightIdString = string(char(signalLightId));

== matlab function EV_longitude/RealSim/MATLAB Function ==
  data: strUint8Vec input; intVal output double; strLen input
function intVal = strVec2Int(strUint8Vec, strLen)

    strVec = blanks(50);
    for i = 1:strLen
       strVec(i) = strUint8Vec(i); 
    end
    if strLen > 0
        intVal = real(str2double(strVec(1:strLen)));
    else
        intVal = -1;
    end
